simulink model "StateMachine"  (R2020b)
settings: Solver=FixedStepAuto  StartTime=0.0  StopTime=40  FixedStep=1  RelTol=1e-3
undefined symbols (not defined in the file): sigbuilder_block
settings Model: EnablePacing=on  PacingRate=1000  Creator=Shubham  LastModifiedBy=Shubham
settings DataIOCC: ExternalInput=[time, levels]

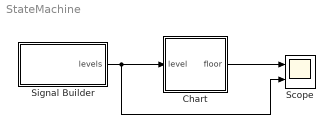
== system StateMachine ==
  Chart : Stateflow chart  TreatAsAtomicUnit=on
  Scope : Scope  NumInputPorts=2
  Signal Builder : Subsystem  Tag=STV Subsys  LoadFcn=sigbuilder_block('load');  StartFcn=sigbuilder_block('start');  StopFcn=sigbuilder_block('stop');  ClipboardFcn=sigbuilder_block('clipboard');  mask(Sigbuilder block){tuvar=[0:10]}
      mask help: Simulink:masks:SigbuilderBlock_MD
      mask init:
      | if ~strcmp(get_param(bdroot(gcbh),'SimulationStatus'),'stopped') tuvar = sigbuilder_block('maskInit'); end
      settings: CopyFcn=sigbuilder_block('copy');  DeleteFcn=sigbuilder_block('delete');  ModelCloseFcn=sigbuilder_block('modelClose');  PreSaveFcn=sigbuilder_block('preSave');  PauseFcn=sigbuilder_block('pause');  ContinueFcn=sigbuilder_block('continue');  NameChangeFcn=sigbuilder_block('namechange');  OpenFcn=sigbuilder_block('open',[0.6 30.6 574.8 555.6 ]);  CloseFcn=sigbuilder_block('close');
      mask Display: plot(0, 0, 100, 100,[2, 2, 32, 32, 2], [68, 8, 8, 68, 68],[32, 2], [38, 38], [32, 19, 2],[53, 60, 44], [32, 17, 17, 2],[16, 16, 31, 31]);txt = getActiveGroup(gcbh);text(2, 100, txt,'verticalAlignment', 'top');
  wires:
  Chart/1(floor) -> Scope/1
  Signal Builder/1(levels) -> Scope/2, Chart/1(level)

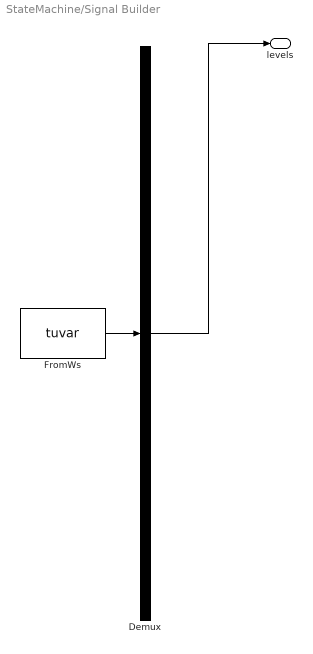
== system StateMachine/Signal Builder ==
  Demux : Demux  Tag=STV Demux  Outputs=1
      settings: DisplayOption=none
  FromWs : FromWorkspace  Tag=STV FromWs  VariableName=tuvar
      SigBuilderData=|
      | common.afterFinalStr = 'Extrapolate'
      | common.sampleTime = 0
      | dataSet.timeRange = [0 40]
      | dataSet.name = 'Sheet1'
      | sbobj.Groups.Name = 'Sheet1'
      | sbobj.Groups.Signals.Name = 'levels'
      | sbobj.Groups.Signals.XData = [0 6 6 10 10 18 18 25 25 30 30 40]
      | sbobj.Groups.Signals.YData = [3 3 5 5 2 2 4 4 1 1 5 5]
      | sbobj.Groups.TimeRange = [0 28]
  levels : Outport  Tag=STV Outport
  wires:
  Demux/1 -> levels/1
  FromWs/1 -> Demux/1

== stateflow chart StateMachine/Chart ==
  state First_Floor
    en:
    floor = 1;
  state Second_Floor
    en:
    floor = 2;
  state Third_Floor
    en:
    floor = 3;
  state Fourth_Floor
    en:
    floor = 4;
  state Fifth_Floor
    en:
    floor = 5;
  (default) -> First_Floor : {floor = 1;}
  Second_Floor -> First_Floor [order 1] : [level < floor]
  First_Floor -> Second_Floor : [level > floor]
  Third_Floor -> Second_Floor [order 1] : [level < floor]
  Second_Floor -> Third_Floor [order 2] : [level > floor]
  Fourth_Floor -> Third_Floor [order 1] : [level < floor]
  Third_Floor -> Fourth_Floor [order 2] : [level > floor]
  Fifth_Floor -> Fourth_Floor : [level < floor]
  Fourth_Floor -> Fifth_Floor [order 2] : [level > floor]
  data: level input; floor output
